simulink model "simulacion"  (R2023b)
settings: Solver=VariableStepAuto  StartTime=0.0  StopTime=10  RelTol=1e-3
values from neighbouring files (symbols this model uses):
  load_voltage_den = [C_L*R_L 1]    [Copy_of_script_1.m]    (also in Variables.m)
  load_voltage_num = R_L    (= 10)    [Copy_of_script_1.m]    (also in Variables.m)
  sys_b_den = [L_b R_b]    [Copy_of_script_1.m]    (also in Variables.m)
  sys_b_num = 1    [Copy_of_script_1.m]    (also in Variables.m)
  sys_fc_den = [L_fc R_fc]    [Copy_of_script_1.m]    (also in Variables.m)
  sys_fc_num = 1    [Copy_of_script_1.m]    (also in Variables.m)
settings Model: Creator=Admin  LastModifiedBy=gonza
settings ModelReferenceCC: EnableRefExpFcnMdlSchedulingChecks=on

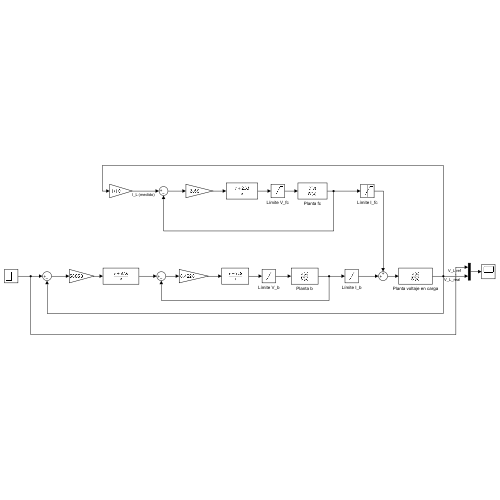
[thumbnail: Simulink's stored preview of the top-level diagram]
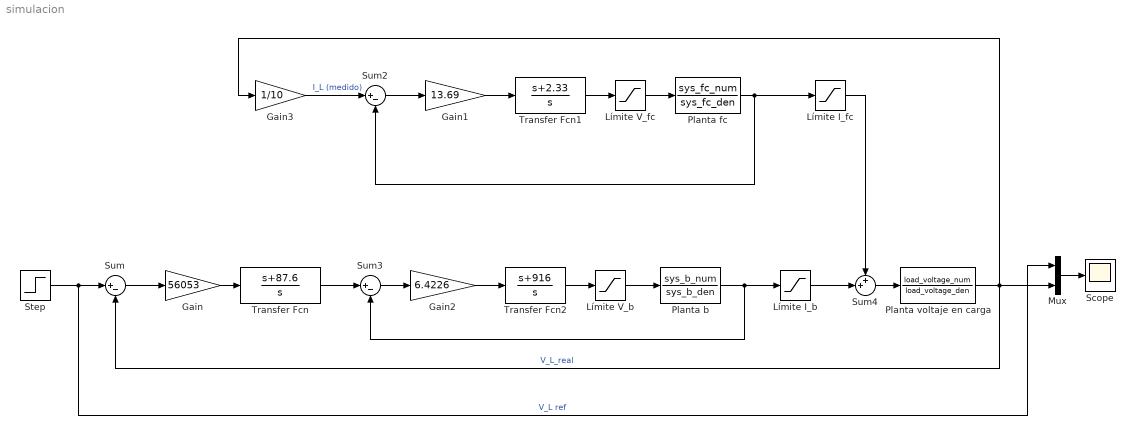
== system simulacion ==
  Gain : Gain  Gain=56053
  Gain1 : Gain  Gain=13.69
  Gain2 : Gain  Gain=6.4226
  Gain3 : Gain  Gain=1/10
  Límite I_b : Saturate  UpperLimit=120  LowerLimit=-120
  Límite I_fc : Saturate  UpperLimit=200  LowerLimit=0
  Límite V_b : Saturate  UpperLimit=400  LowerLimit=-400
  Límite V_fc : Saturate  UpperLimit=450  LowerLimit=0
  Mux : Mux  Inputs=2
  Planta b : TransferFcn  Numerator=sys_b_num  Denominator=sys_b_den
  Planta fc : TransferFcn  Numerator=sys_fc_num  Denominator=sys_fc_den
  Planta voltaje en carga : TransferFcn  Numerator=load_voltage_num  Denominator=load_voltage_den
  Scope : Scope
  Step : Step  After=250  SampleTime=0
  Sum : Sum  Inputs=|+-
  Sum2 : Sum  Inputs=|+-
  Sum3 : Sum  Inputs=|+-
  Sum4 : Sum  Inputs=++|
  Transfer Fcn : TransferFcn  Numerator=[1 87.6]  Denominator=[1 0]
  Transfer Fcn1 : TransferFcn  Numerator=[1 2.33]  Denominator=[1 0]
  Transfer Fcn2 : TransferFcn  Numerator=[1 916]  Denominator=[1 0]
  wires:
  Step/1 -> Mux/1, Sum/1  "V_L ref"
  Sum/1 -> Gain/1
  Gain/1 -> Transfer Fcn/1
  Transfer Fcn/1 -> Sum3/1
  Sum3/1 -> Gain2/1
  Gain2/1 -> Transfer Fcn2/1
  Transfer Fcn2/1 -> Límite V_b/1
  Sum4/1 -> Planta voltaje en carga/1
  Planta voltaje en carga/1 -> Gain3/1, Sum/2, Mux/2  "V_L_real"
  Mux/1 -> Scope/1
  Límite I_b/1 -> Sum4/2
  Planta b/1 -> Límite I_b/1, Sum3/2
  Límite V_b/1 -> Planta b/1
  Límite I_fc/1 -> Sum4/1
  Gain1/1 -> Transfer Fcn1/1
  Gain3/1 -> Sum2/1  "I_L (medido)"
  Transfer Fcn1/1 -> Límite V_fc/1
  Límite V_fc/1 -> Planta fc/1
  Sum2/1 -> Gain1/1
  Planta fc/1 -> Límite I_fc/1, Sum2/2
